simulink model "Calculator"  (R2016b)
settings: Solver=FixedStepDiscrete  StartTime=0.0  StopTime=10.0  RelTol=1e-3
settings Model: Creator=Dell  LastModifiedBy=Dell
settings OptimizationCC: DefaultParameterBehavior=Inlined
settings DebuggingCC: ParameterTunabilityLossMsg=error
settings RTWCC: SystemTargetFile=ert.tlc  TemplateMakefile=ert_default_tmf  Description=Embedded Coder  GenerateReport=on  IncludeHyperlinkInReport=on  LaunchReport=on  GenerateTraceInfo=on  GenerateTraceReport=on  GenerateTraceReportSl=on  GenerateTraceReportSf=on  GenerateTraceReportEml=on
settings CodeAppCC: ForceParamTrailComments=on  IgnoreCustomStorageClasses=off  OperatorAnnotations=on  SimulinkDataObjDesc=on  SFDataObjDesc=on  MATLABFcnDesc=on  InsertBlockDesc=on  MATLABSourceComments=on
settings ERTTargetCC: TargetLangStandard=C99 (ISO)  GenerateSampleERTMain=on  InlinedParameterPlacement=NonHierarchical  ERTCustomFileTemplate=example_file_process.tlc

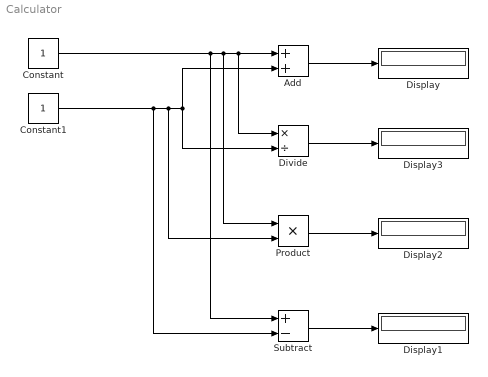
== system Calculator ==
  Add : Sum
  Constant : Constant
  Constant1 : Constant
  Display{,1..3} (4 alike) : Display
  Divide : Product  Inputs=*/
  Product : Product
  Subtract : Sum  Inputs=+-
  wires:
  Constant/1 -> Subtract/1, Product/1, Divide/1, Add/1
  Constant1/1 -> Subtract/2, Product/2, Divide/2, Add/2
  Add/1 -> Display/1
  Divide/1 -> Display3/1
  Product/1 -> Display2/1
  Subtract/1 -> Display1/1
